simulink model "PenduloInvertido_TCC"  (R2020a)
settings: Solver=FixedStepDiscrete  StartTime=0.0  StopTime=30  FixedStep=0.02  RelTol=1e-3  EnableMultiTasking=on
libraries: RASPlib x4
settings Model: SILPILModeSetting=veronly  ExtModeTrigDuration=2  Creator=mathe  LastModifiedBy=mathe
settings OptimizationCC: EnhancedBackFolding=on  PassReuseOutputArgsAs=Individual arguments  ZeroExternalMemoryAtStartup=off  ZeroInternalMemoryAtStartup=off  MaxStackSize=64  OptimizeBlockOrder=speed  DifferentSizesBufferReuse=on  OptimizationCustomize=off  EfficientTunableParamExpr=on
settings DebuggingCC: ParameterTunabilityLossMsg=error
settings HardwareCC: ProdBitPerInt=16  ProdBitPerPointer=16  ProdBitPerSizeT=16  ProdBitPerPtrDiffT=16  ProdLargestAtomicFloat=None  ProdWordSize=8  ProdHWDeviceType=Atmel->AVR  UseEmbeddedCoderFeatures=off
settings SFSimCC: MATLABDynamicMemAlloc=off
settings RTWCC: SystemTargetFile=ert.tlc  HardwareBoard=Arduino Mega 2560  TLCOptions=-aInlineSetEventsForThisBaseRateFcn=TLC_FALSE -aSuppressMultiTaskScheduler=TLC_FALSE -aRateBasedStepFcn=1  TemplateMakefile=ert_default_tmf  Toolchain=Arduino AVR  BuildConfiguration=Faster Runs
settings CodeAppCC: ForceParamTrailComments=on  IgnoreCustomStorageClasses=off  OperatorAnnotations=on  SimulinkDataObjDesc=on  SFDataObjDesc=on  InsertBlockDesc=on
settings ERTTargetCC: SupportContinuousTime=on  SupportNonInlinedSFcns=on  SupportVariableSizeSignals=on  ExtModeStaticAllocSize=2048

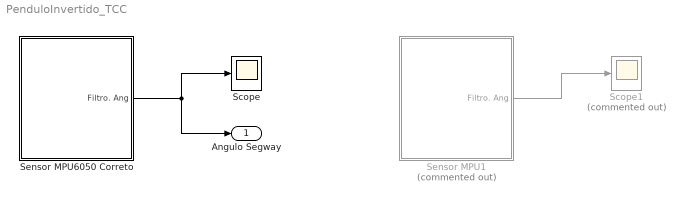
== system PenduloInvertido_TCC ==
  Scope : Scope
  Scope1 : Scope  Commented=on
  Sensor MPU1 : Subsystem  Commented=on
  Sensor MPU6050 Correto : Subsystem
  Angulo Segway : Outport
  wires:
  Sensor MPU1/1(Filtro. Ang) -> Scope1/1
  Sensor MPU6050 Correto/1(Filtro. Ang) -> Scope/1, Angulo Segway/1

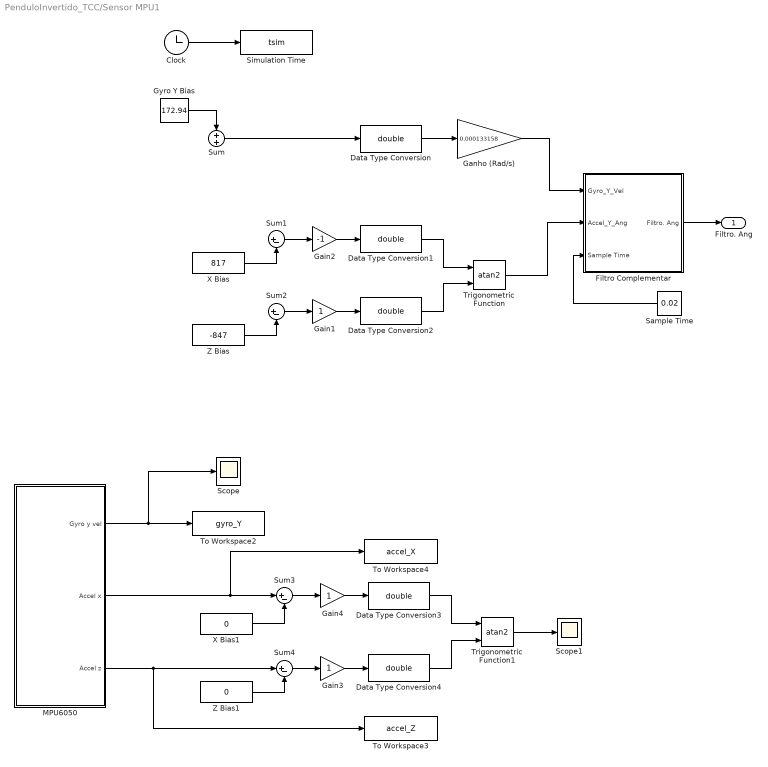
== system PenduloInvertido_TCC/Sensor MPU1 ==
  Clock : Clock
      settings: Decimation=30
  Data Type Conversion{,1..4} (5 alike) : DataTypeConversion  OutDataTypeStr=double
  Filtro Complementar : Subsystem
  Gain1 : Gain
  Gain2 : Gain  Gain=-1
  Gain3 : Gain
  Gain4 : Gain
  Ganho (Rad/s) : Gain  Gain=0.000133158
  Gyro Y Bias : Constant  Value=172.94
  MPU6050 : Subsystem
  Sample Time : Constant  Value=0.02
  Scope : Scope
  Scope1 : Scope
  Simulation Time : ToWorkspace  VariableName=tsim  SampleTime=-1
  Sum : Sum
  Sum{1..4} (4 alike) : Sum  Inputs=|+-
  To Workspace2 : ToWorkspace  VariableName=gyro_Y  SampleTime=-1
      settings: Save2DSignal=2-D array (concatenate along first dimension)
  To Workspace3 : ToWorkspace  VariableName=accel_Z  SampleTime=-1
      settings: Save2DSignal=2-D array (concatenate along first dimension)
  To Workspace4 : ToWorkspace  VariableName=accel_X  SampleTime=-1
      settings: Save2DSignal=2-D array (concatenate along first dimension)
  Trigonometric Function : Trigonometry  Operator=atan2
  Trigonometric Function1 : Trigonometry  Operator=atan2
  X Bias : Constant  Value=817
  X Bias1 : Constant  Value=0
  Z Bias : Constant  Value=-847
  Z Bias1 : Constant  Value=0
  Filtro. Ang : Outport
  wires:
  Data Type Conversion1/1 -> Trigonometric Function/1
  Sample Time/1 -> Filtro Complementar/3(Sample Time)
  Gyro Y Bias/1 -> Sum/1
  Data Type Conversion2/1 -> Trigonometric Function/2
  Trigonometric Function/1 -> Filtro Complementar/2(Accel_Y_Ang)
  Data Type Conversion/1 -> Ganho (Rad/s)/1
  Filtro Complementar/1(Filtro. Ang) -> Filtro. Ang/1
  X Bias/1 -> Sum1/2
  Z Bias/1 -> Sum2/2
  Sum2/1 -> Gain1/1
  Gain1/1 -> Data Type Conversion2/1
  Sum1/1 -> Gain2/1
  Gain2/1 -> Data Type Conversion1/1
  Clock/1 -> Simulation Time/1
  MPU6050/1(Gyro y vel) -> To Workspace2/1, Scope/1
  MPU6050/2(Accel x) -> To Workspace4/1, Sum3/1
  MPU6050/3(Accel z) -> To Workspace3/1, Sum4/1
  Sum/1 -> Data Type Conversion/1
  Ganho (Rad/s)/1 -> Filtro Complementar/1(Gyro_Y_Vel)
  Gain3/1 -> Data Type Conversion4/1
  Gain4/1 -> Data Type Conversion3/1
  Sum3/1 -> Gain4/1
  Data Type Conversion4/1 -> Trigonometric Function1/2
  X Bias1/1 -> Sum3/2
  Data Type Conversion3/1 -> Trigonometric Function1/1
  Sum4/1 -> Gain3/1
  Z Bias1/1 -> Sum4/2
  Trigonometric Function1/1 -> Scope1/1

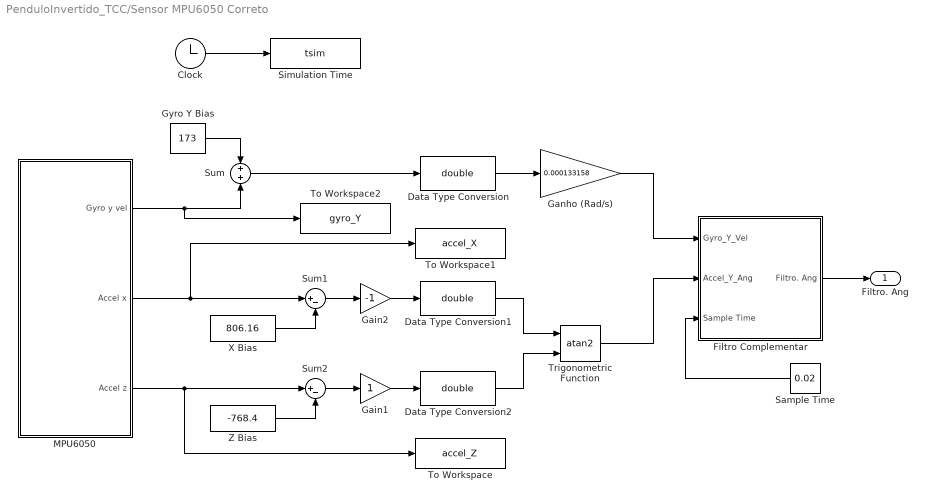
== system PenduloInvertido_TCC/Sensor MPU6050 Correto ==
  Clock : Clock
      settings: Decimation=30
  Data Type Conversion : DataTypeConversion  OutDataTypeStr=double
  Data Type Conversion1 : DataTypeConversion  OutDataTypeStr=double
  Data Type Conversion2 : DataTypeConversion  OutDataTypeStr=double
  Filtro Complementar : Subsystem
  Gain1 : Gain
  Gain2 : Gain  Gain=-1
  Ganho (Rad/s) : Gain  Gain=0.000133158
  Gyro Y Bias : Constant  Value=173
  MPU6050 : Subsystem
  Sample Time : Constant  Value=0.02
  Simulation Time : ToWorkspace  VariableName=tsim  SampleTime=-1
  Sum : Sum
  Sum1 : Sum  Inputs=|+-
  Sum2 : Sum  Inputs=|+-
  To Workspace : ToWorkspace  VariableName=accel_Z  SampleTime=-1
  To Workspace1 : ToWorkspace  VariableName=accel_X  SampleTime=-1
  To Workspace2 : ToWorkspace  VariableName=gyro_Y  SampleTime=-1
  Trigonometric Function : Trigonometry  Operator=atan2
  X Bias : Constant  Value=806.16
  Z Bias : Constant  Value=-768.4
  Filtro. Ang : Outport
  wires:
  Data Type Conversion1/1 -> Trigonometric Function/1
  Sample Time/1 -> Filtro Complementar/3(Sample Time)
  Sum/1 -> Data Type Conversion/1
  Gyro Y Bias/1 -> Sum/1
  Data Type Conversion2/1 -> Trigonometric Function/2
  MPU6050/1(Gyro y vel) -> To Workspace2/1, Sum/2
  Trigonometric Function/1 -> Filtro Complementar/2(Accel_Y_Ang)
  Data Type Conversion/1 -> Ganho (Rad/s)/1
  Ganho (Rad/s)/1 -> Filtro Complementar/1(Gyro_Y_Vel)
  Filtro Complementar/1(Filtro. Ang) -> Filtro. Ang/1
  X Bias/1 -> Sum1/2
  MPU6050/2(Accel x) -> To Workspace1/1, Sum1/1
  MPU6050/3(Accel z) -> Sum2/1, To Workspace/1
  Z Bias/1 -> Sum2/2
  Sum2/1 -> Gain1/1
  Gain1/1 -> Data Type Conversion2/1
  Sum1/1 -> Gain2/1
  Gain2/1 -> Data Type Conversion1/1
  Clock/1 -> Simulation Time/1

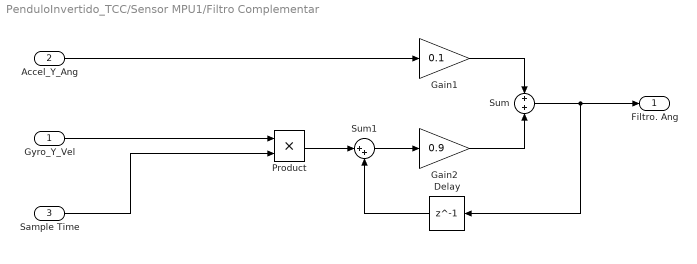
== system PenduloInvertido_TCC/Sensor MPU1/Filtro Complementar ==
  Gyro_Y_Vel : Inport
  Accel_Y_Ang : Inport  Port=2
  Sample Time : Inport  Port=3
  Delay : Delay  DelayLength=1
  Gain1 : Gain  Gain=0.1
  Gain2 : Gain  Gain=0.9
  Product : Product
  Sum : Sum
  Sum1 : Sum  Inputs=|++
  Filtro. Ang : Outport
  wires:
  Delay/1 -> Sum1/2
  Gain1/1 -> Sum/1
  Product/1 -> Sum1/1
  Sum1/1 -> Gain2/1
  Gain2/1 -> Sum/2
  Sample Time/1 -> Product/2
  Gyro_Y_Vel/1 -> Product/1
  Accel_Y_Ang/1 -> Gain1/1
  Sum/1 -> Delay/1, Filtro. Ang/1

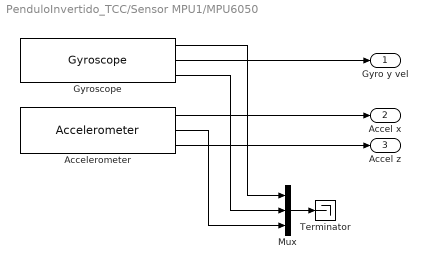
== system PenduloInvertido_TCC/Sensor MPU1/MPU6050 ==
  Accelerometer : RASPlib/Accelerometer  SimulateUsing=Code generation
      settings: SourceProductName=Rensselaer Arduino Support Package
  Gyroscope : RASPlib/Gyroscope  DLPFmode=0
      settings: SourceProductName=Rensselaer Arduino Support Package
  Mux : Mux  Inputs=3
  Terminator : Terminator
  Gyro y vel : Outport
  Accel x : Outport  Port=2
  Accel z : Outport  Port=3
  wires:
  Mux/1 -> Terminator/1
  Gyroscope/2 -> Gyro y vel/1
  Gyroscope/1 -> Mux/1
  Accelerometer/2 -> Mux/3
  Gyroscope/3 -> Mux/2
  Accelerometer/1 -> Accel x/1
  Accelerometer/3 -> Accel z/1

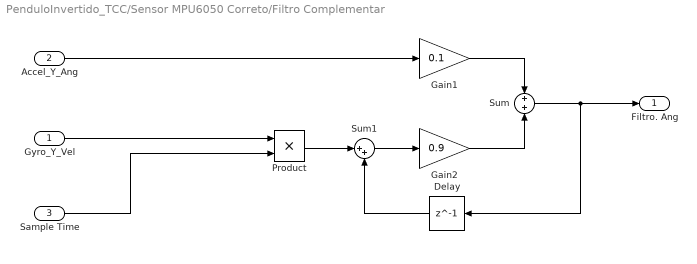
== system PenduloInvertido_TCC/Sensor MPU6050 Correto/Filtro Complementar ==
  Gyro_Y_Vel : Inport
  Accel_Y_Ang : Inport  Port=2
  Sample Time : Inport  Port=3
  Delay : Delay  DelayLength=1
  Gain1 : Gain  Gain=0.1
  Gain2 : Gain  Gain=0.9
  Product : Product
  Sum : Sum
  Sum1 : Sum  Inputs=|++
  Filtro. Ang : Outport
  wires:
  Delay/1 -> Sum1/2
  Gain1/1 -> Sum/1
  Product/1 -> Sum1/1
  Sum1/1 -> Gain2/1
  Gain2/1 -> Sum/2
  Sample Time/1 -> Product/2
  Gyro_Y_Vel/1 -> Product/1
  Accel_Y_Ang/1 -> Gain1/1
  Sum/1 -> Delay/1, Filtro. Ang/1

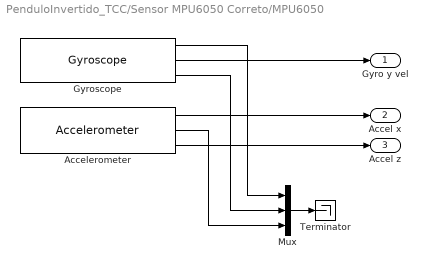
== system PenduloInvertido_TCC/Sensor MPU6050 Correto/MPU6050 ==
  Accelerometer : RASPlib/Accelerometer  SimulateUsing=Code generation
      settings: SourceProductName=Rensselaer Arduino Support Package
  Gyroscope : RASPlib/Gyroscope  DLPFmode=0
      settings: SourceProductName=Rensselaer Arduino Support Package
  Mux : Mux  Inputs=3
  Terminator : Terminator
  Gyro y vel : Outport
  Accel x : Outport  Port=2
  Accel z : Outport  Port=3
  wires:
  Mux/1 -> Terminator/1
  Gyroscope/2 -> Gyro y vel/1
  Gyroscope/1 -> Mux/1
  Accelerometer/2 -> Mux/3
  Gyroscope/3 -> Mux/2
  Accelerometer/1 -> Accel x/1
  Accelerometer/3 -> Accel z/1
